simulink model "ModeloEmBaseNova"  (Simulink 7.1)
settings: Solver=ode45  StartTime=0.0  StopTime=10.0  RelTol=1e-3
values from neighbouring files (symbols this model uses):
  A_ = Q * A * inv(Q)    [BaseNova.m]
  B_ = Q * B    [BaseNova.m]
  C_ = [C * inv(Q); 1 0 0; 0 1 0; 0 0 1]    [BaseNova.m]
settings Model: Creator=ALUNO  LastModifiedBy=ALUNO

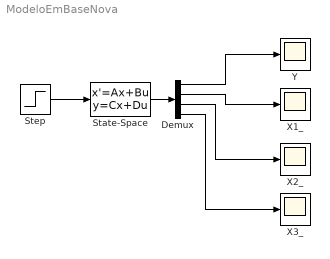
== system ModeloEmBaseNova ==
  Demux : Demux
  State-Space : StateSpace  A=A_  B=B_  C=C_  D=[0;0;0;0]
  Step : Step  Time=0  SampleTime=0
  X1_ : Scope
  X2_ : Scope
      settings: SaveName=ScopeData2
  X3_ : Scope
      settings: SaveName=ScopeData3
  Y : Scope
  wires:
  Step/1 -> State-Space/1
  State-Space/1 -> Demux/1
  Demux/1 -> Y/1
  Demux/2 -> X1_/1
  Demux/3 -> X2_/1
  Demux/4 -> X3_/1
